simulink model "problem1model"  (R2020a)
settings: Solver=VariableStepAuto  StartTime=0.0  StopTime=10.0  RelTol=1e-3
PostLoadFcn:
  | K1=50;
  | M1=100;
  | K12=200;
  | M2=2;
  | t=10;
  | B=50;
settings Model: Creator=Jake  LastModifiedBy=Jake

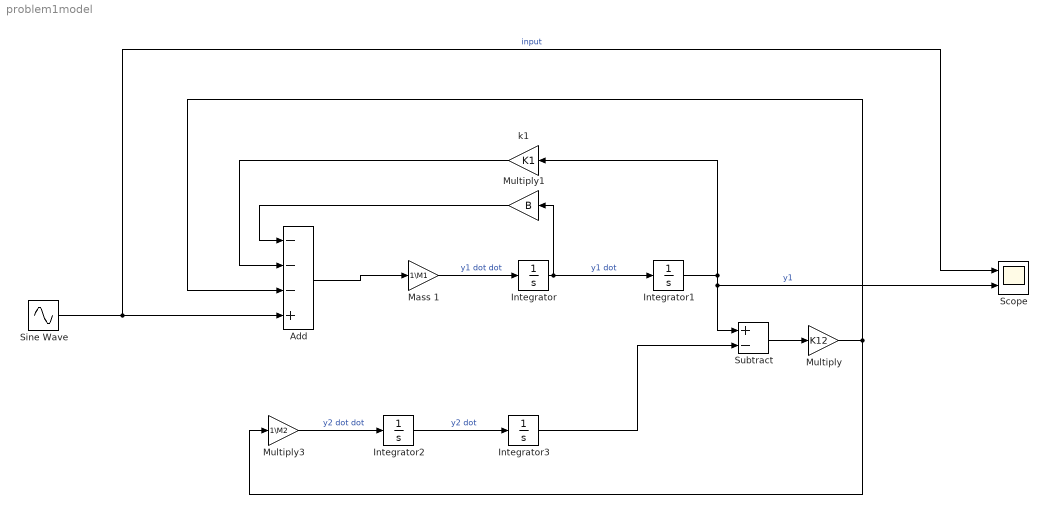
== system problem1model ==
  Add : Sum  Inputs=---+
  Integrator{,1..3} (4 alike) : Integrator
  Mass 1 : Gain  Gain=1\M1
  Multiply : Gain  Gain=K12
  Multiply1 : Gain  Gain=B
  Multiply3 : Gain  Gain=1\M2
  Scope : Scope  NumInputPorts=2
  Sine Wave : Sin  Amplitude=2*sin(10*t)  SampleTime=0
  Subtract : Sum  Inputs=+-
  k1 : Gain  Gain=K1
  wires:
  Mass 1/1 -> Integrator/1  "y1 dot dot"
  Integrator/1 -> Multiply1/1, Integrator1/1  "y1 dot"
  Integrator1/1 -> Scope/2, Subtract/1, k1/1  "y1"
  k1/1 -> Add/2
  Add/1 -> Mass 1/1
  Multiply1/1 -> Add/1
  Multiply3/1 -> Integrator2/1  "y2 dot dot"
  Integrator2/1 -> Integrator3/1  "y2 dot"
  Integrator3/1 -> Subtract/2
  Subtract/1 -> Multiply/1
  Multiply/1 -> Multiply3/1, Add/3
  Sine Wave/1 -> Scope/1, Add/4  "input"
